simulink model "SistemaCompleto_PMSM"  (R2023b)
settings: Solver=VariableStepAuto  StartTime=0.0  StopTime=2  RelTol=1e-3
PostLoadFcn:
  | parametros_sistema_completo
  | run("parametros_sistema_completo.mlx")
values from neighbouring files (symbols this model uses):
  a_cu = 3.9e-3    (= 0.0039)    [parametros_sistema_completo.m]    (also in workspace_params.mat)
  A_i = [0,  1,                          0 ... (first row only)    [analisis_estabilidad_LA.m]
  b_eq = params.b_total    [calcular_matriz_AO.m]    (also in calculo_incertidumbre_y_control.m = b_m + b_l/(r^2); parametros_sistema_completo.m = 2.19444444444e-05; workspace_params.mat = 2.19444444444e-05)
  C_ts = C_ts * (1 + tol_pct)    [calculo_incertidumbre_y_control.m]    (also in parametros_sistema_completo.m = 0.818; workspace_params.mat = 0.818)
  g = 9.80665    [parametros_sistema_completo.m]    (also in workspace_params.mat)
  J_eq = params.J_total    [calcular_matriz_AO.m]    (also in calculo_incertidumbre_y_control.m = J_m + J_l/r^2; parametros_sistema_completo.m = 1.97847222222e-05; workspace_params.mat = 3.28055555556e-05)
  k_l = m*l_cm + m_l*l_l    [calculo_incertidumbre_y_control.m]    (also in parametros_sistema_completo.m = 0.25; workspace_params.mat = 0.625)
  L_d = L_d    * (1 - tol_pct)    [calculo_incertidumbre_y_control.m]    (also in parametros_sistema_completo.m = 0.0066; workspace_params.mat = 0.0066)
  L_ls = L_ls   * (1 - tol_pct)    [calculo_incertidumbre_y_control.m]    (also in parametros_sistema_completo.m = 0.0008; workspace_params.mat = 0.0008)
  L_q = L_q    * (1 - tol_pct)    [calculo_incertidumbre_y_control.m]    (also in parametros_sistema_completo.m = 0.0058; workspace_params.mat = 0.0058)
  lambda_r = lambda_r * (1 + tol_pct)    [calculo_incertidumbre_y_control.m]    (also in parametros_sistema_completo.m = 0.016; workspace_params.mat = 0.016)
  P_p = 3    [parametros_sistema_completo.m]    (also in workspace_params.mat)
  params = struct()    [evaluar_migracion_Ids.m]    (also in parametros_sistema_completo.m; workspace_params.mat = )
  r = params.r_red    [calcular_matriz_AO.m]    (also in parametros_sistema_completo.m = 120; workspace_params.mat = 120)
  R_s_sim = R_sREF * (1 + a_cu * (T_s_sim - T_sREF))    [configurar_temperatura_516.m]
  R_sREF = R_sREF * (1 - tol_pct)    [calculo_incertidumbre_y_control.m]    (also in parametros_sistema_completo.m = 1.02; workspace_params.mat = 1.02)
  R_ts_amb = R_ts_amb * (1 - tol_pct)    [calculo_incertidumbre_y_control.m]    (also in parametros_sistema_completo.m = 146.7; workspace_params.mat = 146.7)
  T_amb = 20    [parametros_sistema_completo.m]    (also in workspace_params.mat)
  T_s = x(6)    [modulador_torque_521.m]    (also in simulacion_dinamica_516.m)
  T_sREF = 20    [parametros_sistema_completo.m]    (also in workspace_params.mat)
undefined symbols (not defined in the file or in its folder): A_T, A_theta, A_v, b_a, B_i, B_T, B_theta, B_v, C_i, C_T, C_theta, C_v, consigna_posicion, D_i, D_T, D_theta, D_v, i_ds_inicial, Is_pico, Is_rms_max, Is_rms_nom, K_e_i_m_int, K_e_tita_m, K_e_tita_m_int, K_e_w_m, K_e_w_m_int, K_p0, K_pd, K_pq, K_sa, K_sia, pos_inicial, t_rampa_acel, t_rampa_vel, V_sl_max, x0_ias, x0_ibs, x0_ics, x0_T, x0_theta
libraries: simulink_extras x8, SignalEditorBlockLib x6, eeStairGenerator x4, simulink x1
(part 6 of 7)

== system SistemaCompleto_PMSM/Modelo Global NL perfil trapezoidal aceleracion2/Planta/Transformacion de Park ==
  f_a : Inport
  f_b : Inport  Port=2
  f_c : Inport  Port=3
  θ_r : Inport  Port=4
  Add : Sum  Inputs=+++
  Add1 : Sum  Inputs=+-
  Add2 : Sum
  Add3 : Sum  Inputs=+++
  Add4 : Sum  Inputs=+++
  Constant : Constant  Value=2/3*pi
  Constant1 : Constant  Value=2/3*pi
  Cos : Trigonometry  Operator=cos
  Cos1 : Trigonometry  Operator=cos
  Cos2 : Trigonometry  Operator=cos
  Cos3 : Trigonometry
  Cos4 : Trigonometry
  Cos5 : Trigonometry
  Gain1 : Gain  Gain=2/3
  Gain2 : Gain  Gain=2/3
  Gain3 : Gain  Gain=1/3
  Product{,1..5} (6 alike) : Product
  f_q : Outport
  f_d : Outport  Port=2
  f_0 : Outport  Port=3
  wires:
  Product4/1 -> Add3/2
  Cos1/1 -> Product1/1
  Cos/1 -> Product/1
  Product1/1 -> Add/2
  Gain1/1 -> f_d/1
  Add3/1 -> Gain1/1
  Cos3/1 -> Product3/1
  Gain3/1 -> f_0/1
  Product2/1 -> Add/3
  Product3/1 -> Add3/1
  Add4/1 -> Gain3/1
  Add2/1 -> Cos5/1, Cos2/1
  f_b/1 -> Add4/2, Product4/2, Product1/2
  Constant1/1 -> Add2/2
  Constant/1 -> Add1/2
  f_c/1 -> Add4/1, Product5/2, Product2/2
  Add1/1 -> Cos4/1, Cos1/1
  Product/1 -> Add/1
  f_a/1 -> Product/2, Product3/2, Add4/3
  Cos2/1 -> Product2/1
  Cos4/1 -> Product4/1
  θ_r/1 -> Add2/1, Add1/1, Cos/1, Cos3/1
  Add/1 -> Gain2/1
  Product5/1 -> Add3/3
  Gain2/1 -> f_q/1
  Cos5/1 -> Product5/1

== system SistemaCompleto_PMSM/Modelo Global NL Retroalimentado/Planta/Subsistema Electromagnetico ==
  v_qs : Inport
  v_ds : Inport  Port=2
  v_0s : Inport  Port=3
  ωm : Inport  Port=4
  R_s : Inport  Port=5
  Add : Sum  Inputs=-++
  Add1 : Sum  Inputs=--+
  Add2 : Sum  Inputs=|-+
  Add3 : Sum  Inputs=|++
  Gain : Gain  Gain=1/L_q
  Gain1 : Gain  Gain=1/L_d
  Gain2 : Gain  Gain=1/L_ls
  Gain3 : Gain  Gain=P_p
  Gain4 : Gain  Gain=L_d
  Gain5 : Gain  Gain=L_q
  Gain6 : Gain  Gain=3/2*P_p
  Gain7 : Gain  Gain=L_d-L_q
  Integrator : Integrator
  Integrator1 : Integrator  InitialCondition=i_ds_inicial
  Integrator2 : Integrator
  Product{,1..6} (7 alike) : Product
  Sum3 : Sum  Inputs=|++
  λ : Constant  Value=lambda_r
  i_qs : Outport
  i_ds : Outport  Port=2
  i_0s : Outport  Port=3
  T_m : Outport  Port=4
  wires:
  v_0s/1 -> Add2/2
  Gain5/1 -> Add/3
  Gain3/1 -> Product4/2, Product3/1  "ωr"
  Integrator/1 -> Product4/1, Product/2, i_qs/1, Product5/1, Product6/1
  v_qs/1 -> Add1/3
  R_s/1 -> Product2/2, Product1/1, Product/1
  Gain4/1 -> Sum3/1
  Product1/1 -> Add/1
  Integrator2/1 -> i_0s/1, Product2/1
  Sum3/1 -> Product3/2
  Integrator1/1 -> Gain4/1, Product1/2, i_ds/1, Product6/2
  Product/1 -> Add1/2
  Product4/1 -> Gain5/1
  ωm/1 -> Gain3/1
  Add3/1 -> Gain6/1
  Gain/1 -> Integrator/1
  Gain6/1 -> T_m/1
  Product2/1 -> Add2/1
  λ/1 -> Sum3/2, Product5/2
  Gain1/1 -> Integrator1/1
  Add/1 -> Gain1/1
  Add1/1 -> Gain/1
  Product6/1 -> Gain7/1
  Product3/1 -> Add1/1
  Gain2/1 -> Integrator2/1
  Gain7/1 -> Add3/2
  v_ds/1 -> Add/2
  Add2/1 -> Gain2/1
  Product5/1 -> Add3/1

== system SistemaCompleto_PMSM/Modelo Global NL Retroalimentado/Planta/Subsistema Mecanico ==
  Tld(t)[N.m] : Inport
  Tm(t)[N.m] : Inport  Port=2
  1/J_eq[kg.m2] : Gain  Gain=1/J_eq
  Gain : Gain  Gain=1/r
  Gain1 : Gain  Gain=1/r
  Integrator : Integrator
  Integrator1 : Integrator
  Sin : Trigonometry
  Sum : Sum  Inputs=-+-
  Sum1 : Sum
  "[N.m/rad]" : Gain  Gain=g*k_l
  b_eq[N.m/rad/s] : Gain  Gain=b_eq
  θm(t) : Outport
  ωm(t) : Outport  Port=2
  wires:
  Gain1/1 -> Sin/1
  Sin/1 -> "[N.m/rad]"/1  "θm[rad]"
  Integrator1/1 -> Integrator/1, ωm(t)/1, b_eq[N.m/rad/s]/1  "ωm[rad/s]"
  Tld(t)[N.m]/1 -> Sum1/1
  b_eq[N.m/rad/s]/1 -> Sum/3
  1/J_eq[kg.m2]/1 -> Integrator1/1  "dω/dt [rad/s^2]"
  Gain/1 -> Sum/1
  "[N.m/rad]"/1 -> Sum1/2
  Integrator/1 -> θm(t)/1, Gain1/1  "θm[rad]"
  Sum/1 -> 1/J_eq[kg.m2]/1
  Tm(t)[N.m]/1 -> Sum/2
  Sum1/1 -> Gain/1

== system SistemaCompleto_PMSM/Modelo Global NL Retroalimentado/Planta/Subsistema Térmico ==
  i_qs2 : Inport
  i_ds2 : Inport  Port=2
  i_0s2 : Inport  Port=3
  Add : Sum  Inputs=+-
  Add1 : Sum
  Add2 : Sum  Inputs=+++
  Add3 : Sum  Inputs=+-
  Add4 : Sum  Inputs=-+
  Constant : Constant  Value=T_sREF
  Constant1 : Constant
  Constant2 : Constant  Value=T_amb
  Gain : Gain  Gain=R_sREF
  Gain1 : Gain  Gain=a_cu
  Gain2 : Gain  Gain=3/2
  Gain3 : Gain  Gain=2
  Gain4 : Gain  Gain=1/C_ts
  Gain5 : Gain  Gain=1/R_ts_amb
  Integrator : Integrator  InitialCondition=T_amb  ZeroCross=off
  Product : Product
  Square : Math  Operator=square  OutDataTypeStr=double
  Square1 : Math  Operator=square
  Square2 : Math  Operator=square
  R_s : Outport
  T_s : Outport  Port=2
  wires:
  Constant1/1 -> Add1/2
  Constant/1 -> Add/2
  i_qs2/1 -> Square/1
  Gain/1 -> R_s/1, Product/1
  Square/1 -> Add2/1
  Add2/1 -> Gain2/1
  Constant2/1 -> Add4/1
  i_ds2/1 -> Square1/1
  Gain5/1 -> Add3/2
  Integrator/1 -> Add4/2, T_s/1, Add/1  "T_s"
  Add1/1 -> Gain/1
  i_0s2/1 -> Square2/1
  Square1/1 -> Add2/2
  Product/1 -> Add3/1  "Ps_Perd"
  Gain2/1 -> Product/2
  Add/1 -> Gain1/1
  Square2/1 -> Gain3/1
  Gain1/1 -> Add1/1
  Add3/1 -> Gain4/1
  Add4/1 -> Gain5/1
  Gain3/1 -> Add2/3
  Gain4/1 -> Integrator/1

== system SistemaCompleto_PMSM/Modelo Global NL Retroalimentado/Planta/TI de Park ==
  f_q : Inport
  f_d : Inport  Port=2
  f_0 : Inport  Port=3
  θ_r : Inport  Port=4
  Add : Sum  Inputs=+++
  Add1 : Sum  Inputs=+-
  Add2 : Sum
  Add3 : Sum  Inputs=+++
  Add4 : Sum  Inputs=+++
  Constant : Constant  Value=2/3*pi
  Constant1 : Constant  Value=2/3*pi
  Cos : Trigonometry  Operator=cos
  Cos1 : Trigonometry
  Cos2 : Trigonometry  Operator=cos
  Cos3 : Trigonometry  Operator=cos
  Cos4 : Trigonometry
  Cos5 : Trigonometry
  Product{,1..5} (6 alike) : Product
  f_a : Outport
  f_b : Outport  Port=2
  f_c : Outport  Port=3
  wires:
  Product4/1 -> Add3/2
  Cos1/1 -> Product1/1
  Cos/1 -> Product/1
  Product1/1 -> Add/2
  Add3/1 -> f_b/1
  Cos3/1 -> Product3/1
  Product3/1 -> Add3/1
  f_d/1 -> Product1/2, Product5/2, Product4/2
  Constant1/1 -> Add2/2
  Constant/1 -> Add1/2
  f_0/1 -> Add3/3, Add4/3, Add/3
  Add1/1 -> Cos3/1, Cos4/1
  Product/1 -> Add/1
  f_q/1 -> Product/2, Product2/2, Product3/2
  Cos4/1 -> Product4/1
  θ_r/1 -> Add2/1, Add1/1, Cos/1, Cos1/1
  Add/1 -> f_a/1
  Add4/1 -> f_c/1
  Cos2/1 -> Product2/1
  Cos5/1 -> Product5/1
  Add2/1 -> Cos5/1, Cos2/1
  Product2/1 -> Add4/1
  Product5/1 -> Add4/2

== system SistemaCompleto_PMSM/Modelo Global NL Retroalimentado/Planta/Transformacion de Park ==
  f_a : Inport
  f_b : Inport  Port=2
  f_c : Inport  Port=3
  θ_r : Inport  Port=4
  Add : Sum  Inputs=+++
  Add1 : Sum  Inputs=+-
  Add2 : Sum
  Add3 : Sum  Inputs=+++
  Add4 : Sum  Inputs=+++
  Constant : Constant  Value=2/3*pi
  Constant1 : Constant  Value=2/3*pi
  Cos : Trigonometry  Operator=cos
  Cos1 : Trigonometry  Operator=cos
  Cos2 : Trigonometry  Operator=cos
  Cos3 : Trigonometry
  Cos4 : Trigonometry
  Cos5 : Trigonometry
  Gain1 : Gain  Gain=2/3
  Gain2 : Gain  Gain=2/3
  Gain3 : Gain  Gain=1/3
  Product{,1..5} (6 alike) : Product
  f_q : Outport
  f_d : Outport  Port=2
  f_0 : Outport  Port=3
  wires:
  Cos5/1 -> Product5/1
  Gain2/1 -> f_q/1
  Product5/1 -> Add3/3
  Add/1 -> Gain2/1
  θ_r/1 -> Cos3/1, Cos/1, Add1/1, Add2/1
  Cos4/1 -> Product4/1
  Cos2/1 -> Product2/1
  f_a/1 -> Add4/3, Product3/2, Product/2
  Product/1 -> Add/1
  Add1/1 -> Cos1/1, Cos4/1
  f_c/1 -> Product2/2, Product5/2, Add4/1
  Constant/1 -> Add1/2
  Constant1/1 -> Add2/2
  f_b/1 -> Product1/2, Product4/2, Add4/2
  Add2/1 -> Cos2/1, Cos5/1
  Add4/1 -> Gain3/1
  Product3/1 -> Add3/1
  Product2/1 -> Add/3
  Gain3/1 -> f_0/1
  Cos3/1 -> Product3/1
  Add3/1 -> Gain1/1
  Gain1/1 -> f_d/1
  Product1/1 -> Add/2
  Cos/1 -> Product/1
  Cos1/1 -> Product1/1
  Product4/1 -> Add3/2

== matlab function SistemaCompleto_PMSM/Modelo Global NL perfil trapezoidal aceleracion y codificado/Controlador/Observador de Estado de velocidad /MATLAB Function ==
  data: theta input; wm_est output; Te_ref input; params input; theta_est output
function [wm_est, theta_est] = observadorEstado(theta, Te_ref, params)
% Observador discreto de velocidad y posicion
% Implementacion equivalente al modelo en bloques con integradores Tustin.
%
% Entradas:
%   theta   : posicion medida [rad]
%   Te_ref  : torque electromagnetico de referencia [N.m]
%   params  : estructura de parametros del controlador
%
% Salidas:
%   wm_est    : velocidad estimada [rad/s]
%   theta_est : posicion estimada [rad]

% =========================
% Lectura de parametros
% =========================
Ts = params.Ts;
J_eq = params.J_eq;

K_e_i_m_int    = params.K_e_i_m_int;
K_e_w_m_int    = params.K_e_w_m_int;
K_e_tita_m_int = params.K_e_tita_m_int;

% =========================
% Estados persistentes
% =========================
persistent theta_est_k wm_est_k
persistent e_prev e_int_prev
persistent dw_prev dtheta_prev

if isempty(theta_est_k)

    theta_est_k = 0;
    wm_est_k    = 0;

    e_prev      = 0;
    e_int_prev  = 0;

    dw_prev     = 0;
    dtheta_prev = 0;
end

% =========================
% Error de posicion
% =========================
e = theta - theta_est_k;

% =========================
% Integrador Tustin del error
% Bloque: Integrador Tustin2
% =========================
e_int = e_int_prev + (Ts/2)*(e + e_prev);

% =========================
% Dinamica de velocidad estimada
% =========================
dw = (1/J_eq)*Te_ref ...
   + K_e_i_m_int*e_int ...
   + K_e_w_m_int*e;

% =========================
% Integrador Tustin de velocidad
% Bloque: Integrador Tustin1
% =========================
wm_est_new = wm_est_k + (Ts/2)*(dw + dw_prev);

% =========================
% Dinamica de posicion estimada
% =========================
dtheta = wm_est_new + K_e_tita_m_int*e;

% =========================
% Integrador Tustin de posicion
% Bloque: Integrador Tustin3
% =========================
theta_est_new = theta_est_k + (Ts/2)*(dtheta + dtheta_prev);

% =========================
% Salidas
% =========================
wm_est    = wm_est_new;
theta_est = theta_est_new;

% =========================
% Actualizacion de estados
% =========================
theta_est_k = theta_est_new;
wm_est_k    = wm_est_new;

e_prev      = e;
e_int_prev  = e_int;

dw_prev     = dw;
dtheta_prev = dtheta;

end

== matlab function SistemaCompleto_PMSM/Modelo Global NL perfil trapezoidal aceleracion y codificado/Controlador/Modulador de Torque/MATLAB Function ==
  data: Tm_ref input; i_qs_ref output; wm input; theta_m input; i_ds input; g input; params input
function i_qs_ref = moduladorTorque(Tm_ref, wm, theta_m, i_ds, g, params)
% Modulador de torque para PMSM.
%
% Calcula la referencia de corriente q:
%
%   i_qs_ref = T_eq / Kt_eq
%
% donde:
%   T_eq  = Tm_ref + b_eq*wm + torque_gravitatorio
%   Kt_eq = (3/2)*Pp*(lambda_m + (Ld - Lq)*i_ds)
%
% Entradas:
%   Tm_ref   : torque mecanico de referencia [N.m]
%   wm       : velocidad mecanica [rad/s]
%   theta_m  : posicion mecanica [rad]
%   i_ds     : corriente eje d [A]
%   g        : gravedad [m/s^2]
%   params   : estructura de parametros
%
% Salida:
%   i_qs_ref : referencia de corriente eje q [A]

% =========================
% Lectura de parametros
% =========================
b_eq     = params.b_eq;
r        = params.r_red;
kl       = params.kl;
Ld       = params.Ld;
Lq       = params.Lq;
Pp       = params.Pp;
lambda_m = params.lambda_m;
Is_pico  = params.Is_pico;

% =========================
% Compensacion viscosa
% =========================
T_visc = b_eq * wm;

% =========================
% Compensacion gravitatoria
% =========================
theta_l = theta_m / r;
T_grav = (kl / r) * sin(theta_l) * g;

% =========================
% Torque equivalente requerido
% =========================
T_eq = Tm_ref + T_visc + T_grav;

% =========================
% Constante de torque equivalente
% =========================
Kt_eq = (3/2) * Pp * (lambda_m + (Ld - Lq) * i_ds);

% =========================
% Calculo de corriente q de referencia
% =========================
i_qs_unsat = T_eq / Kt_eq;

% =========================
% Saturacion entre -Is_pico e Is_pico
% =========================
if i_qs_unsat > Is_pico
    i_qs_ref = Is_pico;
elseif i_qs_unsat < -Is_pico
    i_qs_ref = -Is_pico;
else
    i_qs_ref = i_qs_unsat;
end

end

== matlab function SistemaCompleto_PMSM/Modelo Global NL perfil trapezoidal aceleracion y codificado/Controlador/Modulador de Corriente/MATLAB Function ==
  data: i_qs_ref input; v_qs_ref output; i_qs input; i_ds_ref input; i_ds input; i_0s_ref input; i_0s input; params input; v_ds_ref output; v_0s_ref output
function [v_qs_ref, v_ds_ref, v_0s_ref] = moduladorCorriente(i_qs_ref, i_qs, i_ds_ref, i_ds, i_0s_ref, i_0s, params)
% Modulador de corriente.
% Implementa control proporcional independiente en los ejes q, d y 0.
%
% Entradas:
%   i_qs_ref : referencia de corriente eje q [A]
%   i_qs     : corriente medida eje q [A]
%   i_ds_ref : referencia de corriente eje d [A]
%   i_ds     : corriente medida eje d [A]
%   i_0s_ref : referencia de corriente eje 0 [A]
%   i_0s     : corriente medida eje 0 [A]
%   params   : estructura de parametros
%
% Salidas:
%   v_qs_ref : referencia de tension eje q [V]
%   v_ds_ref : referencia de tension eje d [V]
%   v_0s_ref : referencia de tension eje 0 [V]

% =========================
% Lectura de parametros
% =========================
K_pq = params.K_pq;
K_pd = params.K_pd;
K_p0 = params.K_p0;

% =========================
% Errores de corriente
% =========================
e_iq = i_qs_ref - i_qs;
e_id = i_ds_ref - i_ds;
e_i0 = i_0s_ref - i_0s;

% =========================
% Ley proporcional
% =========================
v_qs_ref = K_pq * e_iq;
v_ds_ref = K_pd * e_id;
v_0s_ref = K_p0 * e_i0;

end

== matlab function SistemaCompleto_PMSM/Modelo Global NL perfil trapezoidal aceleracion y codificado/Controlador/Desacople de Realimentaciones Fisicas Naturales/MATLAB Function ==
  data: v_qs_ref input; v_qs output; Rs input; wm input; v_ds_ref input; v_0s_ref input; i_0s input; i_qs input; i_ds input; params input; v_ds output; v_0s output
function [v_qs, v_ds, v_0s] = desacopleFisico(v_qs_ref, Rs, wm, v_ds_ref, v_0s_ref, i_0s, i_qs, i_ds, params)
% Desacople de realimentaciones fisicas naturales de la PMSM.
%
% Entradas:
%   v_qs_ref : tension q de control [V]
%   Rs       : resistencia estatórica actual [ohm]
%   wm       : velocidad mecanica [rad/s]
%   v_ds_ref : tension d de control [V]
%   v_0s_ref : tension 0 de control [V]
%   i_0s     : corriente eje 0 [A]
%   i_qs     : corriente eje q [A]
%   i_ds     : corriente eje d [A]
%   params   : estructura de parametros
%
% Salidas:
%   v_qs : tension q desacoplada [V]
%   v_ds : tension d desacoplada [V]
%   v_0s : tension 0 desacoplada [V]

% =========================
% Lectura de parametros
% =========================
lambda_m = params.lambda_m;
Ld       = params.Ld;
Lq       = params.Lq;
Pp       = params.Pp;

% =========================
% Terminos de desacople eje q
% =========================
lambda_eq = lambda_m + Ld*i_ds;

v_qs_ff = wm * Pp * lambda_eq;

% =========================
% Terminos de desacople eje d
% =========================
v_ds_ff = -wm * Pp * Lq * i_qs;

% =========================
% Caidas resistivas
% =========================
v_Rq = Rs * i_qs;
v_Rd = Rs * i_ds;
v_R0 = Rs * i_0s;

% =========================
% Tensiones finales
% =========================
v_qs = v_qs_ref + v_Rq + v_qs_ff;
v_ds = v_ds_ref + v_Rd + v_ds_ff;
v_0s = v_0s_ref + v_R0;

end

== matlab function SistemaCompleto_PMSM/Modelo Global NL perfil trapezoidal aceleracion y codificado/Controlador/T. Directa de Park/MATLAB Function ==
  data: f_a input; f_q output; f_b input; f_c input; theta_m input; f_d output; f_0 output; params input
function [f_q, f_d, f_0] = parkDirecta(f_a, f_b, f_c, theta_m, params)

Pp = params.Pp;
theta = Pp * theta_m;

theta_a = theta;
theta_b = theta - 2*pi/3;
theta_c = theta + 2*pi/3;

c_a = cos(theta_a);
c_b = cos(theta_b);
c_c = cos(theta_c);

s_a = sin(theta_a);
s_b = sin(theta_b);
s_c = sin(theta_c);

f_q = (2/3)*(f_a*c_a + f_b*c_b + f_c*c_c);

f_d = -(2/3)*(f_a*s_a + f_b*s_b + f_c*s_c);

f_0 = (1/3)*(f_a + f_b + f_c);

end

== matlab function SistemaCompleto_PMSM/Modelo Global NL perfil trapezoidal aceleracion/MATLAB Function ==
  settings: updateMethod=DISCRETE  sampleTime=1e-4
  data: t input; theta_ref output; omega_ref output; consigna_posicion parameter size=[100 2]; t_rampa_vel parameter; t_rampa_acel parameter; accel_ref output
function [theta_ref,omega_ref,accel_ref]= GeneradorTrayectoria(t,consigna_posicion, t_rampa_vel, t_rampa_acel)
persistent inicializado
persistent dt_vec dq_vec
persistent h1_vec h2_vec
persistent tr1_vec tr2_vec
persistent t_nodos q_nodos N

if isempty(inicializado)
    N = 0;
    for i = 1:size(consigna_posicion,1)
        if ~isnan(consigna_posicion(i,1)) && ~isnan(consigna_posicion(i,2))
            N = N + 1;
        else
            break;
        end
    end

    if N < 2
        error('Debe haber al menos 2 puntos válidos en Matriz_Consigna');
    end
    t_nodos = consigna_posicion(1:N,1);
    q_nodos = consigna_posicion(1:N,2);
    n_tramos = N-1;
    dt_vec = zeros(n_tramos,1);
    dq_vec = zeros(n_tramos,1);
    h1_vec = zeros(n_tramos,1);
    h2_vec = zeros(n_tramos,1);
    tr1_vec = zeros(n_tramos,1);
    tr2_vec = zeros(n_tramos,1);
    for k = 1:n_tramos
        dt_vec(k) = t_nodos(k+1)-t_nodos(k);
        dq_vec(k) = q_nodos(k+1)-q_nodos(k);

        tr1_vec(k)=t_rampa_vel;
        tr2_vec(k)=t_rampa_acel;

        if tr1_vec(k) <= 0
            error('t_rampa_vel debe ser > 0 en el tramo %d.',k);
        end

        if tr2_vec(k) <= 0 || tr2_vec(k) >= tr1_vec(k)
            error('Debe cumplirse 0 < t_rampa_acel < t_rampa_vel en el tramo %d.',k);
        end

        if dt_vec(k) < 2*tr1_vec(k)
            error('Debe cumplirse dt >= 2*t_rampa_vel en el tramo %d.',k);
        end
        %Altura velocidad
        h1_vec(k) = abs(dq_vec(k))/(dt_vec(k)-tr1_vec(k));
        h2_vec(k) = h1_vec(k)/(tr1_vec(k)-tr2_vec(k));
    end
    inicializado=true;
end

if t <= t_nodos(1)
    theta_ref = q_nodos(1);
    omega_ref = 0;
    accel_ref = 0;
    return;
end

if t>= t_nodos(end)
    theta_ref = q_nodos(end);
    omega_ref = 0;
    accel_ref = 0;
    return;
end

tramo_actual = 1;
for k = 1:(N-1)
    if t >= t_nodos(k) && t < t_nodos(k+1)
        tramo_actual = k;
        break;
    end
end
tau = t - t_nodos(tramo_actual);

q0  = q_nodos(tramo_actual);
dt  = dt_vec(tramo_actual);
dq  = dq_vec(tramo_actual);
h1  = h1_vec(tramo_actual);
h2  = h2_vec(tramo_actual);
tr1 = tr1_vec(tramo_actual);
tr2 = tr2_vec(tramo_actual);
sgn = sign(dq);
dq_abs = abs(dq);
if dq_abs < 1e-12
    theta_ref = q0;
    omega_ref = 0;
    accel_ref = 0;
    return;
end

% if tau < tr1
%     % Aceleración
%     omega_ref = h1 * (tau / tr1);
%     theta_ref = q0 + 0.5 * (h1/tr1) * tau^2;
% elseif tau < (dt - tr1)
%     % Velocidad constante
%     omega_ref = h1;
%     theta_ref = q0 ...
%         + 0.5*h1*tr1 ...
%         + h1*(tau - tr1);
%
% elseif tau <= dt
%     % Desaceleración
%     td = tau - (dt - tr1);
%     omega_ref = h1 * (1 - td/tr1);
%     theta_ref = q_nodos(tramo_actual+1) ...
%         - 0.5 * (h1/tr1) * (dt - tau)^2;
% else
%     theta_ref = q_nodos(tramo_actual+1);
%     omega_ref = 0;
% end

[theta_ref, omega_ref, accel_ref] = perfil_7_subtramos( ...
    tau, q0, q_nodos(tramo_actual+1), dt, h1, h2, tr1, tr2, sgn);
end

function [theta_ref, omega_ref, accel_ref] = perfil_7_subtramos(tau, q0, qf, dt, h1, h2, tr1, tr2, sgn)

    d_acc = 0.5*h1*tr1;

    if tau <= 0
        theta_ref = q0;
        omega_ref = 0;
        accel_ref = 0;

    elseif tau < tr1
        [s_local, w_local, a_local] = perfil_arranque_local(tau, h2, tr1, tr2);
        theta_ref = q0 + sgn*s_local;
        omega_ref = sgn*w_local;
        accel_ref = sgn*a_local;

    elseif tau < (dt - tr1)
        u = tau - tr1;
        theta_ref = q0 + sgn*(d_acc + h1*u);
        omega_ref = sgn*h1;
        accel_ref = 0;

    elseif tau <= dt
        rho = dt - tau;
        [s_local, w_local, a_local] = perfil_arranque_local(rho, h2, tr1, tr2);
        theta_ref = qf - sgn*s_local;
        omega_ref = sgn*w_local;
        accel_ref = -sgn*a_local;

    else
        theta_ref = qf;
        omega_ref = 0;
        accel_ref = 0;
    end
end
function [s_local, w_local, a_local] = perfil_arranque_local(tloc, h2, tr1, tr2)

    t1 = tr2;
    t2 = tr1 - tr2;

    if tloc <= 0
        s_local = 0;
        w_local = 0;
        a_local = 0;

    elseif tloc < t1
        % Subtramo 1: aceleración sube linealmente
        a_local = (h2/tr2)*tloc;
        w_local = (h2/(2*tr2))*tloc^2;
        s_local = (h2/(6*tr2))*tloc^3;

    elseif tloc < t2
        % Subtramo 2: aceleración constante = h2
        u = tloc - tr2;

        w1 = h2*tr2/2;
        s1 = h2*tr2^2/6;

        a_local = h2;
        w_local = w1 + h2*u;
        s_local = s1 + w1*u + 0.5*h2*u^2;

    elseif tloc <= tr1
        % Subtramo 3: aceleración baja linealmente hasta 0
        u = tloc - (tr1 - tr2);

        w2 = h2*tr2/2 + h2*(tr1 - 2*tr2);
        s2 = h2*tr2^2/6 ...
           + (h2*tr2/2)*(tr1 - 2*tr2) ...
           + 0.5*h2*(tr1 - 2*tr2)^2;

        a_local = h2 - (h2/tr2)*u;
        w_local = w2 + h2*u - (h2/(2*tr2))*u^2;
        s_local = s2 + w2*u + 0.5*h2*u^2 - (h2/(6*tr2))*u^3;

    else
        a_local = 0;
        w_local = h2*(tr1 - tr2);   % = h1
        s_local = 0.5*w_local*tr1;
    end
end

== matlab function SistemaCompleto_PMSM/Modelo Global NL perfil trapezoidal aceleracion y codificado/Controlador/T. Inversa de Park/MATLAB Function ==
  data: f_q input; f_a output; f_d input; f_0 input; theta_m input; f_b output; f_c output; params input
function [f_a, f_b, f_c] = parkInversa(f_q, f_d, f_0, theta_m, params)

Pp = params.Pp;
theta = Pp * theta_m;

theta_a = theta;
theta_b = theta - 2*pi/3;
theta_c = theta + 2*pi/3;

f_a = f_q*cos(theta_a) - f_d*sin(theta_a) + f_0;
f_b = f_q*cos(theta_b) - f_d*sin(theta_b) + f_0;
f_c = f_q*cos(theta_c) - f_d*sin(theta_c) + f_0;

end

== matlab function SistemaCompleto_PMSM/Modelo Global NL Retroalimentado/MATLAB Function2 ==
  data: Vas input; delta_deg output; Vbs input; Vcs input; theta_m input; vqs_ref input
function delta_deg = anguloCarga(Vas, Vbs, Vcs, theta_m, vqs_ref)
    Pp = 3;
    theta_r = Pp * theta_m;

    v_qs =  (2/3)*( Vas*cos(theta_r) + Vbs*cos(theta_r-2*pi/3) + Vcs*cos(theta_r+2*pi/3) );
    v_ds = -(2/3)*( Vas*sin(theta_r) + Vbs*sin(theta_r-2*pi/3) + Vcs*sin(theta_r+2*pi/3) );

    if abs(vqs_ref) < 1
        delta_deg = 0;
        return;
    end

    s = sign(vqs_ref);                 % sentido de la tensión q
    delta = atan2(v_ds*s, v_qs*s);     % desfasaje respecto al eje q activo
    delta_deg = delta * 180/pi;
end

== matlab function SistemaCompleto_PMSM/Modelo Global /MATLAB Function ==
  settings: updateMethod=DISCRETE
  data: theta_ev output; theta input; theta_prev input; vueltas_actuales input; vueltas_nuevas output
function [theta_ev,vueltas_nuevas]  = phase_unwrap(theta,theta_prev,vueltas_actuales)

delta_theta = theta-theta_prev;

if delta_theta > pi
    vueltas_nuevas = vueltas_actuales - 1;
elseif delta_theta < -pi
    vueltas_nuevas = vueltas_actuales + 1;
else
    vueltas_nuevas = vueltas_actuales;
end
theta_ev = theta + 2*pi*vueltas_nuevas;
end

== matlab function SistemaCompleto_PMSM/Modelo Global NL Controlador modulador de torque3/MATLAB Function ==
  settings: updateMethod=DISCRETE  sampleTime=1e-4
  data: t input; theta_ref output; omega_ref output; consigna_posicion parameter size=[20 2]; t_rampa_vel parameter; t_rampa_acel parameter; accel_ref output
function [theta_ref,omega_ref,accel_ref]= GeneradorTrayectoria(t,consigna_posicion, t_rampa_vel, t_rampa_acel)
persistent inicializado
persistent dt_vec dq_vec
persistent h1_vec h2_vec
persistent tr1_vec tr2_vec
persistent t_nodos q_nodos N

if isempty(inicializado)
    N = 0;
    for i = 1:size(consigna_posicion,1)
        if ~isnan(consigna_posicion(i,1)) && ~isnan(consigna_posicion(i,2))
            N = N + 1;
        else
            break;
        end
    end

    if N < 2
        error('Debe haber al menos 2 puntos válidos en Matriz_Consigna');
    end
    t_nodos = consigna_posicion(1:N,1);
    q_nodos = consigna_posicion(1:N,2);
    n_tramos = N-1;
    dt_vec = zeros(n_tramos,1);
    dq_vec = zeros(n_tramos,1);
    h1_vec = zeros(n_tramos,1);
    h2_vec = zeros(n_tramos,1);
    tr1_vec = zeros(n_tramos,1);
    tr2_vec = zeros(n_tramos,1);
    for k = 1:n_tramos
        dt_vec(k) = t_nodos(k+1)-t_nodos(k);
        dq_vec(k) = q_nodos(k+1)-q_nodos(k);

        tr1_vec(k)=t_rampa_vel;
        tr2_vec(k)=t_rampa_acel;

        if tr1_vec(k) <= 0
            error('t_rampa_vel debe ser > 0 en el tramo %d.',k);
        end

        if tr2_vec(k) <= 0 || tr2_vec(k) >= tr1_vec(k)
            error('Debe cumplirse 0 < t_rampa_acel < t_rampa_vel en el tramo %d.',k);
        end

        if dt_vec(k) < 2*tr1_vec(k)
            error('Debe cumplirse dt >= 2*t_rampa_vel en el tramo %d.',k);
        end
        %Altura velocidad
        h1_vec(k) = abs(dq_vec(k))/(dt_vec(k)-tr1_vec(k));
        h2_vec(k) = h1_vec(k)/(tr1_vec(k)-tr2_vec(k));
    end
    inicializado=true;
end

if t <= t_nodos(1)
    theta_ref = q_nodos(1);
    omega_ref = 0;
    accel_ref = 0;
    return;
end

if t>= t_nodos(end)
    theta_ref = q_nodos(end);
    omega_ref = 0;
    accel_ref = 0;
    return;
end

tramo_actual = 1;
for k = 1:(N-1)
    if t >= t_nodos(k) && t < t_nodos(k+1)
        tramo_actual = k;
        break;
    end
end
tau = t - t_nodos(tramo_actual);

q0  = q_nodos(tramo_actual);
dt  = dt_vec(tramo_actual);
dq  = dq_vec(tramo_actual);
h1  = h1_vec(tramo_actual);
h2  = h2_vec(tramo_actual);
tr1 = tr1_vec(tramo_actual);
tr2 = tr2_vec(tramo_actual);
sgn = sign(dq);
dq_abs = abs(dq);
if dq_abs < 1e-12
    theta_ref = q0;
    omega_ref = 0;
    accel_ref = 0;
    return;
end

% if tau < tr1
%     % Aceleración
%     omega_ref = h1 * (tau / tr1);
%     theta_ref = q0 + 0.5 * (h1/tr1) * tau^2;
% elseif tau < (dt - tr1)
%     % Velocidad constante
%     omega_ref = h1;
%     theta_ref = q0 ...
%         + 0.5*h1*tr1 ...
%         + h1*(tau - tr1);
%
% elseif tau <= dt
%     % Desaceleración
%     td = tau - (dt - tr1);
%     omega_ref = h1 * (1 - td/tr1);
%     theta_ref = q_nodos(tramo_actual+1) ...
%         - 0.5 * (h1/tr1) * (dt - tau)^2;
% else
%     theta_ref = q_nodos(tramo_actual+1);
%     omega_ref = 0;
% end

[theta_ref, omega_ref, accel_ref] = perfil_7_subtramos( ...
    tau, q0, q_nodos(tramo_actual+1), dt, h1, h2, tr1, tr2, sgn);
end

function [theta_ref, omega_ref, accel_ref] = perfil_7_subtramos(tau, q0, qf, dt, h1, h2, tr1, tr2, sgn)

    d_acc = 0.5*h1*tr1;

    if tau <= 0
        theta_ref = q0;
        omega_ref = 0;
        accel_ref = 0;

    elseif tau < tr1
        [s_local, w_local, a_local] = perfil_arranque_local(tau, h2, tr1, tr2);
        theta_ref = q0 + sgn*s_local;
        omega_ref = sgn*w_local;
        accel_ref = sgn*a_local;

    elseif tau < (dt - tr1)
        u = tau - tr1;
        theta_ref = q0 + sgn*(d_acc + h1*u);
        omega_ref = sgn*h1;
        accel_ref = 0;

    elseif tau <= dt
        rho = dt - tau;
        [s_local, w_local, a_local] = perfil_arranque_local(rho, h2, tr1, tr2);
        theta_ref = qf - sgn*s_local;
        omega_ref = sgn*w_local;
        accel_ref = -sgn*a_local;

    else
        theta_ref = qf;
        omega_ref = 0;
        accel_ref = 0;
    end
end
function [s_local, w_local, a_local] = perfil_arranque_local(tloc, h2, tr1, tr2)

    t1 = tr2;
    t2 = tr1 - tr2;

    if tloc <= 0
        s_local = 0;
        w_local = 0;
        a_local = 0;

    elseif tloc < t1
        % Subtramo 1: aceleración sube linealmente
        a_local = (h2/tr2)*tloc;
        w_local = (h2/(2*tr2))*tloc^2;
        s_local = (h2/(6*tr2))*tloc^3;

    elseif tloc < t2
        % Subtramo 2: aceleración constante = h2
        u = tloc - tr2;

        w1 = h2*tr2/2;
        s1 = h2*tr2^2/6;

        a_local = h2;
        w_local = w1 + h2*u;
        s_local = s1 + w1*u + 0.5*h2*u^2;

    elseif tloc <= tr1
        % Subtramo 3: aceleración baja linealmente hasta 0
        u = tloc - (tr1 - tr2);

        w2 = h2*tr2/2 + h2*(tr1 - 2*tr2);
        s2 = h2*tr2^2/6 ...
           + (h2*tr2/2)*(tr1 - 2*tr2) ...
           + 0.5*h2*(tr1 - 2*tr2)^2;

        a_local = h2 - (h2/tr2)*u;
        w_local = w2 + h2*u - (h2/(2*tr2))*u^2;
        s_local = s2 + w2*u + 0.5*h2*u^2 - (h2/(6*tr2))*u^3;

    else
        a_local = 0;
        w_local = h2*(tr1 - tr2);   % = h1
        s_local = 0.5*w_local*tr1;
    end
end

== matlab function SistemaCompleto_PMSM/Modelo Global NL Controlador modulador de torque4/MATLAB Function ==
  settings: updateMethod=DISCRETE  sampleTime=1e-4
  data: t input; theta_ref output; omega_ref output; consigna_posicion parameter size=[20 2]; t_rampa_vel parameter; t_rampa_acel parameter
function [theta_ref,omega_ref]= GeneradorTrayectoria(t,consigna_posicion, t_rampa_vel, t_rampa_acel)
persistent inicializado
persistent dt_vec dq_vec
persistent h1_vec h2_vec
persistent tr1_vec tr2_vec
persistent t_nodos q_nodos N

if isempty(inicializado)
    N = 0;
    for i = 1:size(consigna_posicion,1)
        if ~isnan(consigna_posicion(i,1)) && ~isnan(consigna_posicion(i,2))
            N = N + 1;
        else
            break;
        end
    end

    if N < 2
        error('Debe haber al menos 2 puntos válidos en Matriz_Consigna');
    end
    t_nodos = consigna_posicion(:,1);
    q_nodos = consigna_posicion(:,2);
    n_tramos = N-1;
    dt_vec = zeros(n_tramos,1);
    dq_vec = zeros(n_tramos,1);
    h1_vec = zeros(n_tramos,1);
    h2_vec = zeros(n_tramos,1);
    tr1_vec = zeros(n_tramos,1);
    tr2_vec = zeros(n_tramos,1);
    for k = 1:n_tramos
        dt_vec(k) = t_nodos(k+1)-t_nodos(k);
        dq_vec(k) = q_nodos(k+1)-q_nodos(k);

        tr1_vec(k)=t_rampa_vel;
        tr2_vec(k)=t_rampa_acel;

        if dt_vec(k) <= tr1_vec(k)
            error('El tramo %d no tiene suficiente tiempo para el perfil.',k);
        end
        %Altura velocidad
        h1_vec(k) = dq_vec(k)/(dt_vec(k)-tr1_vec(k));
        h2_vec(k) = h1_vec(k) /(tr1_vec(k)-tr2_vec(k));
    end
    inicializado=true;
end

if t <= t_nodos(1)
    theta_ref = q_nodos(1);
    omega_ref = 0;
    return;
end

if t>= t_nodos(end)
    theta_ref = q_nodos(end);
    omega_ref = 0;
    return;
end

tramo_actual = 1;
for k = 1:(N-1)
    if t >= t_nodos(k) && t < t_nodos(k+1)
        tramo_actual = k;
        break;
    end
end
tau = t - t_nodos(tramo_actual);

q0  = q_nodos(tramo_actual);
dt  = dt_vec(tramo_actual);
dq  = dq_vec(tramo_actual);
h1  = h1_vec(tramo_actual);
h2  = h2_vec(tramo_actual);
tr1 = tr1_vec(tramo_actual);
tr2 = tr2_vec(tramo_actual);

if abs(dq) < 1e-12
    theta_ref = q0;
    omega_ref = 0;
    return;
end

if tau < tr1
    % Aceleración
    omega_ref = h1 * (tau / tr1);
    theta_ref = q0 + 0.5 * (h1/tr1) * tau^2;
elseif tau < (dt - tr1)
    % Velocidad constante
    omega_ref = h1;
    theta_ref = q0 ...
        + 0.5*h1*tr1 ...
        + h1*(tau - tr1);

elseif tau <= dt
    % Desaceleración
    td = tau - (dt - tr1);
    omega_ref = h1 * (1 - td/tr1);
    theta_ref = q_nodos(tramo_actual+1) ...
        - 0.5 * (h1/tr1) * (dt - tau)^2;
else
    theta_ref = q_nodos(tramo_actual+1);
    omega_ref = 0;
end

end

== matlab function SistemaCompleto_PMSM/Modelo Global NL perfil trapezoidal aceleracion1/MATLAB Function ==
  settings: updateMethod=DISCRETE  sampleTime=1e-4
  data: t input; theta_ref output; omega_ref output; consigna_posicion parameter size=[4 2]; t_rampa_vel parameter; t_rampa_acel parameter; accel_ref output
function [theta_ref,omega_ref,accel_ref]= GeneradorTrayectoria(t,consigna_posicion, t_rampa_vel, t_rampa_acel)
persistent inicializado
persistent dt_vec dq_vec
persistent h1_vec h2_vec
persistent tr1_vec tr2_vec
persistent t_nodos q_nodos N

if isempty(inicializado)
    N = 0;
    for i = 1:size(consigna_posicion,1)
        if ~isnan(consigna_posicion(i,1)) && ~isnan(consigna_posicion(i,2))
            N = N + 1;
        else
            break;
        end
    end

    if N < 2
        error('Debe haber al menos 2 puntos válidos en Matriz_Consigna');
    end
    t_nodos = consigna_posicion(1:N,1);
    q_nodos = consigna_posicion(1:N,2);
    n_tramos = N-1;
    dt_vec = zeros(n_tramos,1);
    dq_vec = zeros(n_tramos,1);
    h1_vec = zeros(n_tramos,1);
    h2_vec = zeros(n_tramos,1);
    tr1_vec = zeros(n_tramos,1);
    tr2_vec = zeros(n_tramos,1);
    for k = 1:n_tramos
        dt_vec(k) = t_nodos(k+1)-t_nodos(k);
        dq_vec(k) = q_nodos(k+1)-q_nodos(k);

        tr1_vec(k)=t_rampa_vel;
        tr2_vec(k)=t_rampa_acel;

        if tr1_vec(k) <= 0
            error('t_rampa_vel debe ser > 0 en el tramo %d.',k);
        end

        if tr2_vec(k) <= 0 || tr2_vec(k) >= tr1_vec(k)
            error('Debe cumplirse 0 < t_rampa_acel < t_rampa_vel en el tramo %d.',k);
        end

        if dt_vec(k) < 2*tr1_vec(k)
            error('Debe cumplirse dt >= 2*t_rampa_vel en el tramo %d.',k);
        end
        %Altura velocidad
        h1_vec(k) = abs(dq_vec(k))/(dt_vec(k)-tr1_vec(k));
        h2_vec(k) = h1_vec(k)/(tr1_vec(k)-tr2_vec(k));
    end
    inicializado=true;
end

if t <= t_nodos(1)
    theta_ref = q_nodos(1);
    omega_ref = 0;
    accel_ref = 0;
    return;
end

if t>= t_nodos(end)
    theta_ref = q_nodos(end);
    omega_ref = 0;
    accel_ref = 0;
    return;
end

tramo_actual = 1;
for k = 1:(N-1)
    if t >= t_nodos(k) && t < t_nodos(k+1)
        tramo_actual = k;
        break;
    end
end
tau = t - t_nodos(tramo_actual);

q0  = q_nodos(tramo_actual);
dt  = dt_vec(tramo_actual);
dq  = dq_vec(tramo_actual);
h1  = h1_vec(tramo_actual);
h2  = h2_vec(tramo_actual);
tr1 = tr1_vec(tramo_actual);
tr2 = tr2_vec(tramo_actual);
sgn = sign(dq);
dq_abs = abs(dq);
if dq_abs < 1e-12
    theta_ref = q0;
    omega_ref = 0;
    accel_ref = 0;
    return;
end

% if tau < tr1
%     % Aceleración
%     omega_ref = h1 * (tau / tr1);
%     theta_ref = q0 + 0.5 * (h1/tr1) * tau^2;
% elseif tau < (dt - tr1)
%     % Velocidad constante
%     omega_ref = h1;
%     theta_ref = q0 ...
%         + 0.5*h1*tr1 ...
%         + h1*(tau - tr1);
%
% elseif tau <= dt
%     % Desaceleración
%     td = tau - (dt - tr1);
%     omega_ref = h1 * (1 - td/tr1);
%     theta_ref = q_nodos(tramo_actual+1) ...
%         - 0.5 * (h1/tr1) * (dt - tau)^2;
% else
%     theta_ref = q_nodos(tramo_actual+1);
%     omega_ref = 0;
% end

[theta_ref, omega_ref, accel_ref] = perfil_7_subtramos( ...
    tau, q0, q_nodos(tramo_actual+1), dt, h1, h2, tr1, tr2, sgn);
end

function [theta_ref, omega_ref, accel_ref] = perfil_7_subtramos(tau, q0, qf, dt, h1, h2, tr1, tr2, sgn)

    d_acc = 0.5*h1*tr1;

    if tau <= 0
        theta_ref = q0;
        omega_ref = 0;
        accel_ref = 0;

    elseif tau < tr1
        [s_local, w_local, a_local] = perfil_arranque_local(tau, h2, tr1, tr2);
        theta_ref = q0 + sgn*s_local;
        omega_ref = sgn*w_local;
        accel_ref = sgn*a_local;

    elseif tau < (dt - tr1)
        u = tau - tr1;
        theta_ref = q0 + sgn*(d_acc + h1*u);
        omega_ref = sgn*h1;
        accel_ref = 0;

    elseif tau <= dt
        rho = dt - tau;
        [s_local, w_local, a_local] = perfil_arranque_local(rho, h2, tr1, tr2);
        theta_ref = qf - sgn*s_local;
        omega_ref = sgn*w_local;
        accel_ref = -sgn*a_local;

    else
        theta_ref = qf;
        omega_ref = 0;
        accel_ref = 0;
    end
end
function [s_local, w_local, a_local] = perfil_arranque_local(tloc, h2, tr1, tr2)

    t1 = tr2;
    t2 = tr1 - tr2;

    if tloc <= 0
        s_local = 0;
        w_local = 0;
        a_local = 0;

    elseif tloc < t1
        % Subtramo 1: aceleración sube linealmente
        a_local = (h2/tr2)*tloc;
        w_local = (h2/(2*tr2))*tloc^2;
        s_local = (h2/(6*tr2))*tloc^3;

    elseif tloc < t2
        % Subtramo 2: aceleración constante = h2
        u = tloc - tr2;

        w1 = h2*tr2/2;
        s1 = h2*tr2^2/6;

        a_local = h2;
        w_local = w1 + h2*u;
        s_local = s1 + w1*u + 0.5*h2*u^2;

    elseif tloc <= tr1
        % Subtramo 3: aceleración baja linealmente hasta 0
        u = tloc - (tr1 - tr2);

        w2 = h2*tr2/2 + h2*(tr1 - 2*tr2);
        s2 = h2*tr2^2/6 ...
           + (h2*tr2/2)*(tr1 - 2*tr2) ...
           + 0.5*h2*(tr1 - 2*tr2)^2;

        a_local = h2 - (h2/tr2)*u;
        w_local = w2 + h2*u - (h2/(2*tr2))*u^2;
        s_local = s2 + w2*u + 0.5*h2*u^2 - (h2/(6*tr2))*u^3;

    else
        a_local = 0;
        w_local = h2*(tr1 - tr2);   % = h1
        s_local = 0.5*w_local*tr1;
    end
end

== matlab function SistemaCompleto_PMSM/Modelo Global NL perfil trapezoidal aceleracion2/MATLAB Function ==
  settings: updateMethod=DISCRETE  sampleTime=1e-4
  data: t input; theta_ref output; omega_ref output; consigna_posicion parameter size=[4 2]; t_rampa_vel parameter; t_rampa_acel parameter; accel_ref output
function [theta_ref,omega_ref,accel_ref]= GeneradorTrayectoria(t,consigna_posicion, t_rampa_vel, t_rampa_acel)
persistent inicializado
persistent dt_vec dq_vec
persistent h1_vec h2_vec
persistent tr1_vec tr2_vec
persistent t_nodos q_nodos N

if isempty(inicializado)
    N = 0;
    for i = 1:size(consigna_posicion,1)
        if ~isnan(consigna_posicion(i,1)) && ~isnan(consigna_posicion(i,2))
            N = N + 1;
        else
            break;
        end
    end

    if N < 2
        error('Debe haber al menos 2 puntos válidos en Matriz_Consigna');
    end
    t_nodos = consigna_posicion(1:N,1);
    q_nodos = consigna_posicion(1:N,2);
    n_tramos = N-1;
    dt_vec = zeros(n_tramos,1);
    dq_vec = zeros(n_tramos,1);
    h1_vec = zeros(n_tramos,1);
    h2_vec = zeros(n_tramos,1);
    tr1_vec = zeros(n_tramos,1);
    tr2_vec = zeros(n_tramos,1);
    for k = 1:n_tramos
        dt_vec(k) = t_nodos(k+1)-t_nodos(k);
        dq_vec(k) = q_nodos(k+1)-q_nodos(k);

        tr1_vec(k)=t_rampa_vel;
        tr2_vec(k)=t_rampa_acel;

        if tr1_vec(k) <= 0
            error('t_rampa_vel debe ser > 0 en el tramo %d.',k);
        end

        if tr2_vec(k) <= 0 || tr2_vec(k) >= tr1_vec(k)
            error('Debe cumplirse 0 < t_rampa_acel < t_rampa_vel en el tramo %d.',k);
        end

        if dt_vec(k) < 2*tr1_vec(k)
            error('Debe cumplirse dt >= 2*t_rampa_vel en el tramo %d.',k);
        end
        %Altura velocidad
        h1_vec(k) = abs(dq_vec(k))/(dt_vec(k)-tr1_vec(k));
        h2_vec(k) = h1_vec(k)/(tr1_vec(k)-tr2_vec(k));
    end
    inicializado=true;
end

if t <= t_nodos(1)
    theta_ref = q_nodos(1);
    omega_ref = 0;
    accel_ref = 0;
    return;
end

if t>= t_nodos(end)
    theta_ref = q_nodos(end);
    omega_ref = 0;
    accel_ref = 0;
    return;
end

tramo_actual = 1;
for k = 1:(N-1)
    if t >= t_nodos(k) && t < t_nodos(k+1)
        tramo_actual = k;
        break;
    end
end
tau = t - t_nodos(tramo_actual);

q0  = q_nodos(tramo_actual);
dt  = dt_vec(tramo_actual);
dq  = dq_vec(tramo_actual);
h1  = h1_vec(tramo_actual);
h2  = h2_vec(tramo_actual);
tr1 = tr1_vec(tramo_actual);
tr2 = tr2_vec(tramo_actual);
sgn = sign(dq);
dq_abs = abs(dq);
if dq_abs < 1e-12
    theta_ref = q0;
    omega_ref = 0;
    accel_ref = 0;
    return;
end

% if tau < tr1
%     % Aceleración
%     omega_ref = h1 * (tau / tr1);
%     theta_ref = q0 + 0.5 * (h1/tr1) * tau^2;
% elseif tau < (dt - tr1)
%     % Velocidad constante
%     omega_ref = h1;
%     theta_ref = q0 ...
%         + 0.5*h1*tr1 ...
%         + h1*(tau - tr1);
%
% elseif tau <= dt
%     % Desaceleración
%     td = tau - (dt - tr1);
%     omega_ref = h1 * (1 - td/tr1);
%     theta_ref = q_nodos(tramo_actual+1) ...
%         - 0.5 * (h1/tr1) * (dt - tau)^2;
% else
%     theta_ref = q_nodos(tramo_actual+1);
%     omega_ref = 0;
% end

[theta_ref, omega_ref, accel_ref] = perfil_7_subtramos( ...
    tau, q0, q_nodos(tramo_actual+1), dt, h1, h2, tr1, tr2, sgn);
end

function [theta_ref, omega_ref, accel_ref] = perfil_7_subtramos(tau, q0, qf, dt, h1, h2, tr1, tr2, sgn)

    d_acc = 0.5*h1*tr1;

    if tau <= 0
        theta_ref = q0;
        omega_ref = 0;
        accel_ref = 0;

    elseif tau < tr1
        [s_local, w_local, a_local] = perfil_arranque_local(tau, h2, tr1, tr2);
        theta_ref = q0 + sgn*s_local;
        omega_ref = sgn*w_local;
        accel_ref = sgn*a_local;

    elseif tau < (dt - tr1)
        u = tau - tr1;
        theta_ref = q0 + sgn*(d_acc + h1*u);
        omega_ref = sgn*h1;
        accel_ref = 0;

    elseif tau <= dt
        rho = dt - tau;
        [s_local, w_local, a_local] = perfil_arranque_local(rho, h2, tr1, tr2);
        theta_ref = qf - sgn*s_local;
        omega_ref = sgn*w_local;
        accel_ref = -sgn*a_local;

    else
        theta_ref = qf;
        omega_ref = 0;
        accel_ref = 0;
    end
end
function [s_local, w_local, a_local] = perfil_arranque_local(tloc, h2, tr1, tr2)

    t1 = tr2;
    t2 = tr1 - tr2;

    if tloc <= 0
        s_local = 0;
        w_local = 0;
        a_local = 0;

    elseif tloc < t1
        % Subtramo 1: aceleración sube linealmente
        a_local = (h2/tr2)*tloc;
        w_local = (h2/(2*tr2))*tloc^2;
        s_local = (h2/(6*tr2))*tloc^3;

    elseif tloc < t2
        % Subtramo 2: aceleración constante = h2
        u = tloc - tr2;

        w1 = h2*tr2/2;
        s1 = h2*tr2^2/6;

        a_local = h2;
        w_local = w1 + h2*u;
        s_local = s1 + w1*u + 0.5*h2*u^2;

    elseif tloc <= tr1
        % Subtramo 3: aceleración baja linealmente hasta 0
        u = tloc - (tr1 - tr2);

        w2 = h2*tr2/2 + h2*(tr1 - 2*tr2);
        s2 = h2*tr2^2/6 ...
           + (h2*tr2/2)*(tr1 - 2*tr2) ...
           + 0.5*h2*(tr1 - 2*tr2)^2;

        a_local = h2 - (h2/tr2)*u;
        w_local = w2 + h2*u - (h2/(2*tr2))*u^2;
        s_local = s2 + w2*u + 0.5*h2*u^2 - (h2/(6*tr2))*u^3;

    else
        a_local = 0;
        w_local = h2*(tr1 - tr2);   % = h1
        s_local = 0.5*w_local*tr1;
    end
end
